simulink model "P2_ejer2_a"  (R2023a)
settings: Solver=VariableStepAuto  StartTime=0.0  StopTime=10.0  RelTol=1e-3
InitFcn:
  | N=5;
  | R = 5*N;
  | b= 0.05*N;
  | J = 0.0001;
  | Kt = 0.01*N;
  | Kb = 0.02;
  | L = 2*N;
  | 
  | k1= -4;
  | k2 = -5;
  | k3 = -4;
  | 
  | A = [0,1,0;
  |      0,-b/J,Kt/J;
  |      0,-Kb/L,-R/L];
  | 
  | B = [0;
  |     0;
  |     1/L];
  | 
  | C = [1,0,0;
  |      0,1,0;
  |       0,0,1];
settings Model: Creator=garci  LastModifiedBy=garci

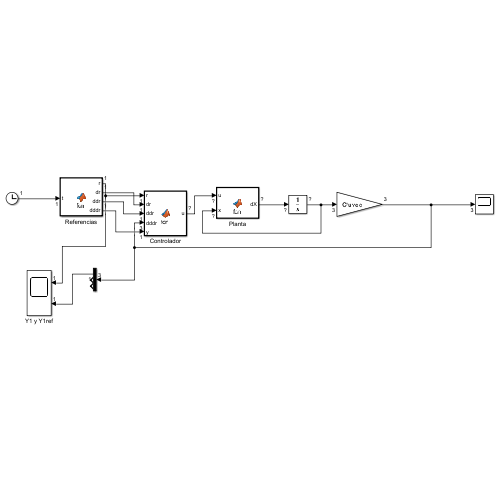
[thumbnail: Simulink's stored preview of the top-level diagram]
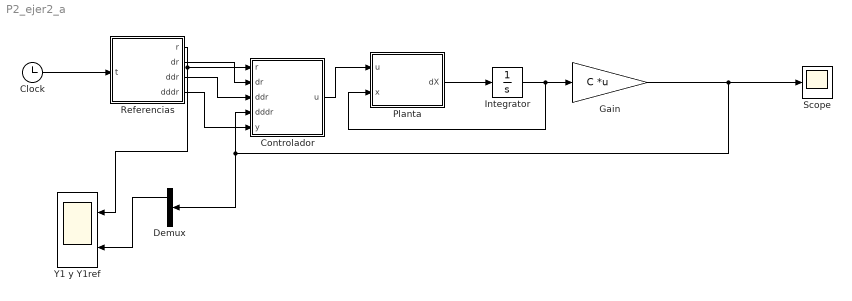
== system P2_ejer2_a ==
  Clock : Clock
  Controlador : MATLAB Function  TreatAsAtomicUnit=on
  Demux : Demux  Outputs=3
  Gain : Gain  Gain=C  Multiplication=Matrix(K*u) (u vector)
  Integrator : Integrator
  Planta : MATLAB Function  TreatAsAtomicUnit=on
  Referencias : MATLAB Function  TreatAsAtomicUnit=on
  Scope : Scope
  Y1 y Y1ref : Scope  NumInputPorts=2
  wires:
  Referencias/1(r) -> Y1 y Y1ref/1, Controlador/1(r)
  Referencias/2(dr) -> Controlador/2(dr)
  Referencias/3(ddr) -> Controlador/3(ddr)
  Controlador/1(u) -> Planta/1(u)
  Planta/1(dX) -> Integrator/1
  Integrator/1 -> Gain/1, Planta/2(x)
  Gain/1 -> Scope/1, Demux/1, Controlador/4(dddr)
  Clock/1 -> Referencias/1(t)
  Referencias/4(dddr) -> Controlador/5(y)
  Demux/1 -> Y1 y Y1ref/2

== matlab function P2_ejer2_a/Controlador ==
  data: r input; u output; dr input; ddr input; dddr input; y input; A parameter; C parameter; k1 parameter; k2 parameter; k3 parameter; b parameter; J parameter; R parameter; L parameter; Kb parameter; Kt parameter
function u = fcn(r,dr,ddr,dddr,y,A,  C,k1, k2, k3, b, J, R, L, Kb, Kt)
%recuperar estados 
X = C^-1 * y;
C1 = C(1,:);
%Primer Bloque
e1 = r - y(1,:);
de1 = dr - C1*(A*X); %Obtener derivada de estado 1 
x2ref = dr - k1*e1;

%Segundo Bloque 
e2 = x2ref - X(2,:); %referencia estado 2 - estado 2

dx2ref = ddr -k1*de1;

de2 = dx2ref - A(2,:)*X;
x3ref = -(k2*e2)/(Kt/J) + ((b/J)/(Kt/J))*A(2,:)*X + dx2ref/(Kt/J); 

%Tercer Bloque
e3 = x3ref - X(3,:);
dx3ref = -k2*de2 + (b/J)*A(2,:)*X + dddr -k1*(ddr - A(2,:)*X);

u = [0;0;L*dx3ref + Kb*X(2,:) + R*X(3,:) - L*k3*e3];

== matlab function P2_ejer2_a/Referencias ==
  data: t input; r output; dr output; ddr output; dddr output; N parameter
function [r,dr,ddr,dddr] = fcn(t,N)

r = 0.5*N + sin(t);
dr = cos(t);
ddr = -sin(t);
dddr = -cos(t);

== matlab function P2_ejer2_a/Planta ==
  data: u input; dX output; A parameter; B parameter; x input
function dX = fcn(u,A, B, x)

dX = A*x + B*u;
